simulink model "motionsim"  (Simulink 10.0)
settings: Solver=ode45  StartTime=0.0  StopTime=200  FixedStep=0.2  RelTol=1e-3  EnableMultiTasking=on
libraries: simulink_extras x3, simulink x1
settings Model: LogicAnalyzerSignalOrdering=bf57a864-7b39-46bb-9a97-b0efb81974cd  Creator=Shao  LastModifiedBy=shao  ExtModeTrigMode=oneshot  ExtModeArmWhenConnect=off
settings SolverCC: ZeroCrossAlgorithm=Adaptive
settings DataIOCC: InspectSignalLogs=on  SignalLoggingName=sigsOut
settings OptimizationCC: BooleanDataType=off
settings DebuggingCC: SaveWithParameterizedLinksMsg=none  SignalResolutionControl=TryResolveAllWithWarning  MultiTaskDSMMsg=warning  MultiTaskCondExecSysMsg=none  StateNameClashWarn=warning
settings HardwareCC: TargetUnknown=on
settings GRTTargetCC: GeneratePreprocessorConditionals=Disable all
settings ConfigComp: CovExternalEMLEnable=off

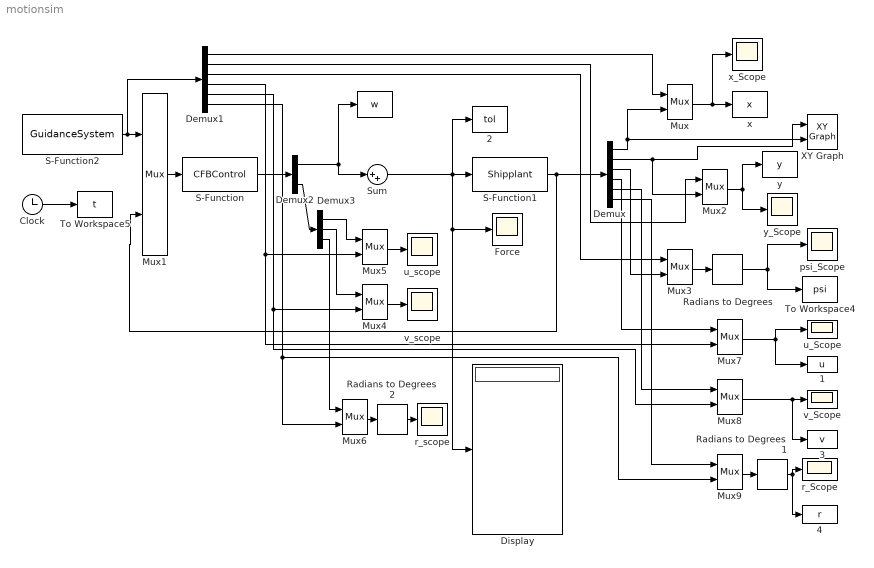
== system motionsim ==
  " " : ToWorkspace  VariableName=w  SampleTime=-1
  " 1" : ToWorkspace  VariableName=u  SampleTime=-1
  " 2" : ToWorkspace  VariableName=tol  SampleTime=-1
  " 3" : ToWorkspace  VariableName=v  SampleTime=-1
  " 4" : ToWorkspace  VariableName=r  SampleTime=-1
  Clock : Clock
  Demux : Demux  Outputs=6
  Demux1 : Demux  Outputs=6
  Demux2 : Demux  Outputs=2
  Demux3 : Demux  Outputs=3
  Display : Display
      settings: Decimation=3
  Force : Scope
  Mux{,1..9} (10 alike) : Mux  Inputs=2
  "Radians to Degrees  " : simulink_extras/Transformations/Radians to Degrees
  Radians to Degrees  1 : simulink_extras/Transformations/Radians to Degrees
  Radians to Degrees  2 : simulink_extras/Transformations/Radians to Degrees
  S-Function : S-Function  FunctionName=CFBControl  SFunctionDeploymentMode=off  EnableBusSupport=off
  S-Function1 : S-Function  FunctionName=Shipplant  SFunctionDeploymentMode=off  EnableBusSupport=off
  S-Function2 : S-Function  FunctionName=GuidanceSystem  SFunctionDeploymentMode=off  EnableBusSupport=off
  Sum : Sum  Inputs=|++
  To Workspace4 : ToWorkspace  VariableName=psi  SampleTime=-1
  To Workspace5 : ToWorkspace  VariableName=t  SampleTime=-1
  XY Graph : simulink/Sinks/XY Graph  xmin=-1  xmax=6  ymin=-1  ymax=5  st=-1
  psi_Scope : Scope
  r_Scope : Scope
  r_scope : Scope
  u_Scope : Scope
  u_scope : Scope
  v_Scope : Scope
  v_scope : Scope
  x : ToWorkspace  VariableName=x  SampleTime=-1
  x_Scope : Scope
  y : ToWorkspace  VariableName=y  SampleTime=-1
  y_Scope : Scope
  wires:
  Mux1/1 -> S-Function/1
  Mux/1 -> x/1, x_Scope/1
  Demux/1 -> Mux/2, XY Graph/2
  S-Function1/1 -> Mux1/2, Demux/1
  Mux2/1 -> y/1, y_Scope/1
  Demux/2 -> XY Graph/1, Mux2/2
  Demux/3 -> Mux3/2
  Clock/1 -> To Workspace5/1
  S-Function2/1 -> Demux1/1, Mux1/1
  Demux1/1 -> Mux/1
  Demux1/2 -> Mux2/1
  Demux1/3 -> Mux3/1
  S-Function/1 -> Demux2/1
  Demux2/1 -> Sum/1, " "/1
  Sum/1 -> " 2"/1, Display/1, Force/1, S-Function1/1
  Mux5/1 -> u_scope/1
  Demux2/2 -> Demux3/1
  Demux3/1 -> Mux5/1
  Demux1/4 -> Mux5/2, Mux7/2
  Mux4/1 -> v_scope/1
  Mux6/1 -> Radians to Degrees  2/1
  Demux3/2 -> Mux4/1
  Demux1/5 -> Mux8/2, Mux4/2
  Demux3/3 -> Mux6/1
  Demux1/6 -> Mux6/2, Mux9/2
  Demux/4 -> Mux7/1
  Demux/5 -> Mux8/1
  Demux/6 -> Mux9/1
  Mux8/1 -> " 3"/1, v_Scope/1
  Mux9/1 -> Radians to Degrees  1/1
  Radians to Degrees  1/1 -> " 4"/1, r_Scope/1
  Mux3/1 -> "Radians to Degrees  "/1
  "Radians to Degrees  "/1 -> To Workspace4/1, psi_Scope/1
  Mux7/1 -> " 1"/1, u_Scope/1
  Radians to Degrees  2/1 -> r_scope/1
